simulink model "justina_ekf"  (R2020a)
settings: Solver=ode4  StartTime=0.0  StopTime=inf  FixedStep=0.004  MaxStep=0.01  RelTol=1e-3
PreLoadFcn:
  | load('justina_rigid_body_tree')
InitFcn:
  | [lowpass_B, lowpass_A] = butter(4,1,'s');
  | manipulator_tree.Gravity = [9.81 0 0];
model workspace (MAT data in the model file):
  SL_ROS_VariableLengthArrays_MaxSizes.CommonInfo.ArrayTruncateAction = 'EmitWarning'
  SL_ROS_VariableLengthArrays_MaxSizes.MsgTypeMap = containers.Map
  SL_ROS_VariableLengthArrays_MaxSizes.MsgTypeMap.serialization.keys = {'sensor_msgs/JointState', 'std_msgs/Float32MultiArray', 'std_msgs/Float64MultiArray', 'std_msgs/String'}
  SL_ROS_VariableLengthArrays_MaxSizes.MsgTypeMap.serialization.values{1}(1).PropertyName = 'Effort'
  SL_ROS_VariableLengthArrays_MaxSizes.MsgTypeMap.serialization.values{1}(1).DataType = 'double'
  SL_ROS_VariableLengthArrays_MaxSizes.MsgTypeMap.serialization.values{1}(1).MaxLength = 7
  SL_ROS_VariableLengthArrays_MaxSizes.MsgTypeMap.serialization.values{1}(2).PropertyName = 'Name'
  SL_ROS_VariableLengthArrays_MaxSizes.MsgTypeMap.serialization.values{1}(2).DataType = 'std_msgs/String'
  SL_ROS_VariableLengthArrays_MaxSizes.MsgTypeMap.serialization.values{1}(2).MaxLength = 7
  SL_ROS_VariableLengthArrays_MaxSizes.MsgTypeMap.serialization.values{1}(3).PropertyName = 'Position'
  SL_ROS_VariableLengthArrays_MaxSizes.MsgTypeMap.serialization.values{1}(3).DataType = 'double'
  SL_ROS_VariableLengthArrays_MaxSizes.MsgTypeMap.serialization.values{1}(3).MaxLength = 7
  SL_ROS_VariableLengthArrays_MaxSizes.MsgTypeMap.serialization.values{1}(4).PropertyName = 'Velocity'
  SL_ROS_VariableLengthArrays_MaxSizes.MsgTypeMap.serialization.values{1}(4).DataType = 'double'
  SL_ROS_VariableLengthArrays_MaxSizes.MsgTypeMap.serialization.values{1}(4).MaxLength = 7
  SL_ROS_VariableLengthArrays_MaxSizes.MsgTypeMap.serialization.values{2}.PropertyName = 'Data'
  SL_ROS_VariableLengthArrays_MaxSizes.MsgTypeMap.serialization.values{2}.DataType = 'single'
  SL_ROS_VariableLengthArrays_MaxSizes.MsgTypeMap.serialization.values{2}.MaxLength = 14
  SL_ROS_VariableLengthArrays_MaxSizes.MsgTypeMap.serialization.values{3}.PropertyName = 'Data'
  SL_ROS_VariableLengthArrays_MaxSizes.MsgTypeMap.serialization.values{3}.DataType = 'double'
  SL_ROS_VariableLengthArrays_MaxSizes.MsgTypeMap.serialization.values{3}.MaxLength = 7
  SL_ROS_VariableLengthArrays_MaxSizes.MsgTypeMap.serialization.values{4}.PropertyName = 'Data'
  SL_ROS_VariableLengthArrays_MaxSizes.MsgTypeMap.serialization.values{4}.DataType = 'uint8'
  SL_ROS_VariableLengthArrays_MaxSizes.MsgTypeMap.serialization.values{4}.MaxLength = 10
  SL_ROS_VariableLengthArrays_MaxSizes.MsgTypeMap.serialization.uniformity = 0
  SL_ROS_VariableLengthArrays_MaxSizes.MsgTypeMap.serialization.keyType = 'char'
  SL_ROS_VariableLengthArrays_MaxSizes.MsgTypeMap.serialization.valueType = 'any'
undefined symbols (not defined in the file or in its folder): Data, Data_SL_Info
libraries: robotlib x6, robotmaniplib x1
settings Model: EnablePacing=on  Creator=marco  LastModifiedBy=josea
settings OptimizationCC: EnhancedBackFolding=on  PassReuseOutputArgsAs=Individual arguments  ZeroExternalMemoryAtStartup=off  ZeroInternalMemoryAtStartup=off  MaxStackSize=64  OptimizeBlockOrder=speed  DifferentSizesBufferReuse=on  OptimizationCustomize=off  EfficientTunableParamExpr=on
settings DebuggingCC: ParameterTunabilityLossMsg=error
settings HardwareCC: ProdBitPerLong=64  ProdHWDeviceType=Intel->x86-64 (Linux 64)
settings SFSimCC: CustomCodeUndefinedFunction=ThrowError
settings RTWCC: SystemTargetFile=ert.tlc  HardwareBoard=Robot Operating System (ROS)  TemplateMakefile=ert_default_tmf  GenerateReport=on  Toolchain=Catkin  IncludeHyperlinkInReport=on  LaunchReport=on  TargetLang=C++  GenerateTraceInfo=on  GenerateTraceReport=on  GenerateTraceReportSl=on  GenerateTraceReportSf=on  GenerateTraceReportEml=on
settings CodeAppCC: ForceParamTrailComments=on  IgnoreCustomStorageClasses=off  OperatorAnnotations=on  SimulinkDataObjDesc=on  SFDataObjDesc=on  InsertBlockDesc=on
settings ERTTargetCC: SupportContinuousTime=on  SupportVariableSizeSignals=on
settings ExplorerConfigSet: InternalSimMechanicsExplorerSettings="<ExplorerConfiguration><canonicalview>aerospace</canonicalview><AnimationSetting><BasePlaybackSpeed>1.0</BasePlaybackSpeed><PlaybackSpeedFactor>1.0</PlaybackSpeedFactor></AnimationSetting><TilePanel><TileInfo><Tiles Columns=\"1\" Count=\"1\" Rows=\"1\"><Column Weight=\"1\"/><Row Weight=\"1\"/><Tile Height=\"1\" Width=\"1\" X=\"0\" Y=\"0\"/></Tiles></TileInfo><SceneInfo><SceneViewer><BGColor><R>0.60000002384185791</R><G>0.60000002384185791</G><B>0.60000002384185791</B></BGColor><Camera><DoPerspective>off</DoPerspective><Position><X>0.470747241724220999</X><Y>0.672742710715300452</Y><Z>0.803552756362765797</Z></Position><Center><X>0.426167977285198674</X><Y>0.0857009724355916047</Y><Z>-0.00477557216445684274</Z></Center><Up><X>-0.998971998504803671</X><Y>0.0328560329609175472</Y><Z>0.0312318315407420499</Z></Up><ViewLimDist>1</ViewLimDist><YLim>0.446111832261085528</YLim><XLim>0.664557689711664734</XLim></Camera></SceneViewer></SceneInfo></TilePanel><MechEditorPanel><Cameras/><GfxPanelCameraMap/><VideoCreator><PlaybackSpeedRatio>1.0</PlaybackSpeedRatio><FrameRate>30</FrameRate><VideoFormat>Motion JPEG AVI</VideoFormat><FrameSize>auto</FrameSize></VideoCreator></MechEditorPanel></ExplorerConfiguration>"

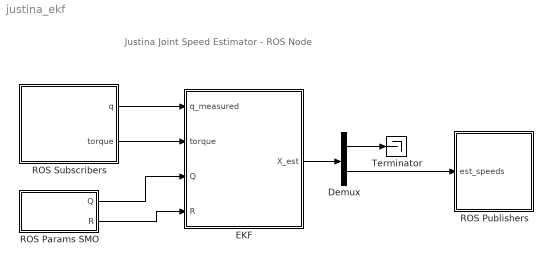
== system justina_ekf ==
  note: Justina Joint Speed Estimator - ROS Node
  Demux : Demux  Outputs=[7,7]
  EKF : Subsystem
  ROS Params SMO : Subsystem
  ROS Publishers : Subsystem
  ROS Subscribers : Subsystem
  Terminator : Terminator
  wires:
  ROS Subscribers/1(q) -> EKF/1(q_measured)
  ROS Subscribers/2(torque) -> EKF/2(torque)
  ROS Params SMO/1(Q) -> EKF/3(Q)
  ROS Params SMO/2(R) -> EKF/4(R)
  Demux/1 -> Terminator/1
  EKF/1(X_est) -> Demux/1
  Demux/2 -> ROS Publishers/1("est_speeds ")

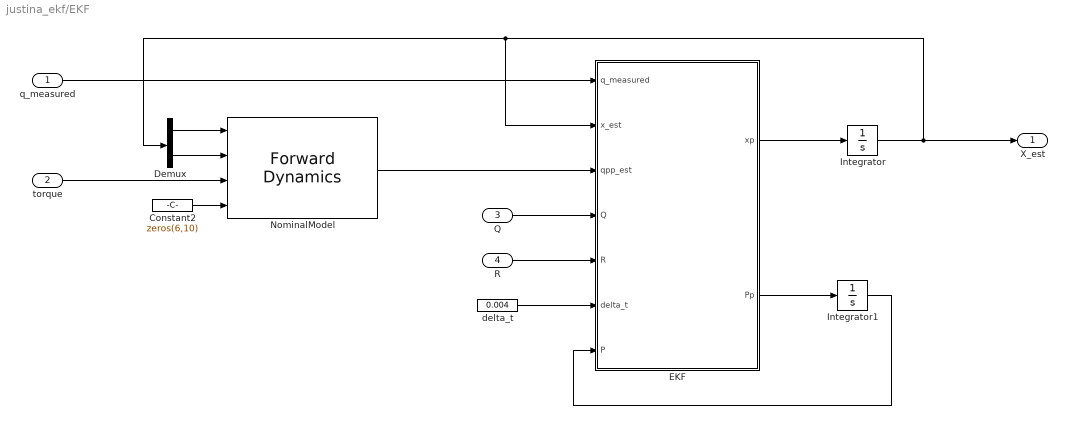
== system justina_ekf/EKF ==
  q_measured : Inport
  torque : Inport  Port=2
  Q : Inport  Port=3
  R : Inport  Port=4
  Constant2 : Constant  Value=zeros(6,10)  SampleTime=-1
  Demux : Demux  Outputs=[7,7]
  EKF : MATLAB Function  TreatAsAtomicUnit=on
  Integrator : Integrator
  Integrator1 : Integrator  InitialCondition=eye(14)*0.001
  NominalModel : robotmaniplib/Forward Dynamics  RigidBodyTree=manipulator_tree  SimulateUsing=Code generation
  delta_t : Constant  Value=0.004  SampleTime=-1
  X_est : Outport
  wires:
  Q/1 -> EKF/4(Q)
  EKF/2(Pp) -> Integrator1/1
  EKF/1(xp) -> Integrator/1
  Constant2/1 -> NominalModel/4
  Demux/2 -> NominalModel/2
  Demux/1 -> NominalModel/1
  delta_t/1 -> EKF/6(delta_t)
  torque/1 -> NominalModel/3
  Integrator1/1 -> EKF/7(P)
  R/1 -> EKF/5(R)
  q_measured/1 -> EKF/1(q_measured)
  Integrator/1 -> X_est/1, EKF/2(x_est), Demux/1
  NominalModel/1 -> EKF/3(qpp_est)

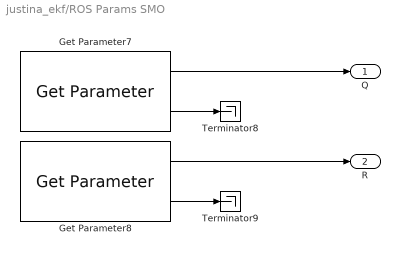
== system justina_ekf/ROS Params SMO ==
  Get Parameter7 : robotlib/Get Parameter  ParameterSource=Specify your own  ParameterName=/ekf/Q  ParameterType=double  ParameterMaxArrayLength=16  ParameterInitialValue=0.0  SampleTime=1  ShowErrorCodeOutput=on  ModelName=ekf  BlockId=ParamGet_ekf_383
      settings: SourceProductBaseCode=RR
  Get Parameter8 : robotlib/Get Parameter  ParameterSource=Specify your own  ParameterName=/ekf/R  ParameterType=double  ParameterMaxArrayLength=16  ParameterInitialValue=0.0  SampleTime=1  ShowErrorCodeOutput=on  ModelName=ekf  BlockId=ParamGet_ekf_384
      settings: SourceProductBaseCode=RR
  Terminator8 : Terminator
  Terminator9 : Terminator
  Q : Outport
  R : Outport  Port=2
  wires:
  Get Parameter7/2 -> Terminator8/1
  Get Parameter7/1 -> Q/1
  Get Parameter8/2 -> Terminator9/1
  Get Parameter8/1 -> R/1

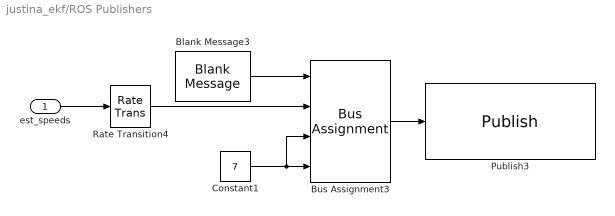
== system justina_ekf/ROS Publishers ==
  "est_speeds " : Inport
  Blank Message3 : robotlib/Blank Message  messageClass=Message  entityType=std_msgs/Float64MultiArray  messageType=std_msgs/Float64MultiArray  SampleTime=0.004
  Bus Assignment3 : BusAssignment  AssignedSignals=Data,Data_SL_Info.CurrentLength,Data_SL_Info.ReceivedLength
  Constant1 : Constant  Value=7  OutDataTypeStr=uint32  SampleTime=0.004
  Publish3 : robotlib/Publish  topicSource=Specify your own  topic=/ekf/estimated_speeds  messageType=std_msgs/Float64MultiArray  messageQueueLength=1
  Rate Transition4 : RateTransition
  wires:
  Rate Transition4/1 -> Bus Assignment3/2
  Bus Assignment3/1 -> Publish3/1
  Constant1/1 -> Bus Assignment3/4, Bus Assignment3/3
  Blank Message3/1 -> Bus Assignment3/1
  "est_speeds "/1 -> Rate Transition4/1

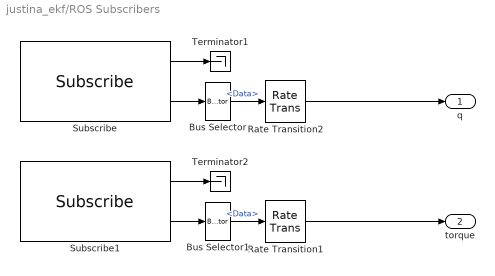
== system justina_ekf/ROS Subscribers ==
  Bus Selector : BusSelector  OutputSignals=Data
  Bus Selector1 : BusSelector  OutputSignals=Data
  Rate Transition1 : RateTransition
  Rate Transition2 : RateTransition
  Subscribe : robotlib/Subscribe  topicSource=Specify your own  topic=/joint_positions  messageType=std_msgs/Float64MultiArray  sampleTime=0.004  messageQueueLength=1
  Subscribe1 : robotlib/Subscribe  topicSource=Specify your own  topic=/joint_torques  messageType=std_msgs/Float64MultiArray  sampleTime=0.004  messageQueueLength=1
  Terminator1 : Terminator
  Terminator2 : Terminator
  q : Outport
  torque : Outport  Port=2
  wires:
  Bus Selector/1 -> Rate Transition2/1  "<Data>"
  Rate Transition2/1 -> q/1
  Subscribe/2 -> Bus Selector/1
  Subscribe/1 -> Terminator1/1
  Subscribe1/1 -> Terminator2/1
  Subscribe1/2 -> Bus Selector1/1
  Bus Selector1/1 -> Rate Transition1/1  "<Data>"
  Rate Transition1/1 -> torque/1

== matlab function justina_ekf/EKF/EKF ==
  data: q_measured input; x_est input; qpp_est input; Q input; R input; delta_t input; P input; xp output; Pp output
function [xp, Pp] = EKF(q_measured, x_est, qpp_est, Q, R, delta_t, P)
xp = zeros(14,1);
e  = zeros(7,1);

Q = Q*eye(14);
R = R*eye(7);

F = [zeros(7,7) eye(7); eye(7)*delta_t eye(7)*delta_t];
H = [eye(7) zeros(7,7)];

K = P*H'/R;
for i=1:7
    xp(i)   = x_est(i+7);
    xp(i+7) = qpp_est(i);
    e(i)    = q_measured(i) - x_est(i);
end
xp = xp + K*e;
Pp = F*P + P*F' - K*R*K' +Q;
